simulink model "dde"  (R2015b)
settings: Solver=ode23s  StartTime=0.0  StopTime=5  RelTol=1e-3
settings Model: Creator=toni  LastModifiedBy=toni
settings DataIOCC: SaveFormat=Array  SignalLoggingSaveFormat=ModelDataLogs  OutputOption=SpecifiedOutputTimes  OutputTimes=[1,2,3,4,5]
settings OptimizationCC: ExpressionDepthLimit=2147483647
settings DebuggingCC: UnderspecifiedInitializationDetection=Classic  MergeDetectMultiDrivingBlocksExec=none  SolverPrmCheckMsg=warning  FcnCallInpInsideContextMsg=EnableAllAsWarning  StateNameClashWarn=warning
settings HardwareCC: ProdBitPerPointer=32  ProdLargestAtomicFloat=None  ProdIntDivRoundTo=Undefined  ProdEndianess=Unspecified  ProdWordSize=32  ProdHWDeviceType=32-bit Generic
settings GRTTargetCC: GeneratePreprocessorConditionals=Disable all
settings ConfigComp: CovModelRefEnable=Off  CovSFcnEnable=off

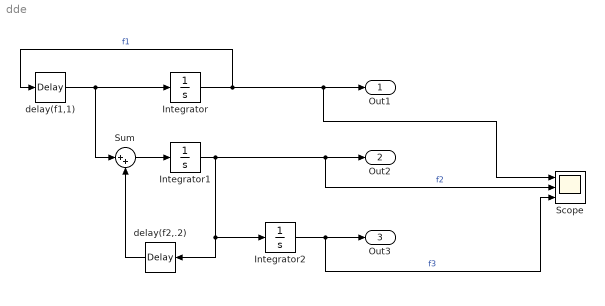
== system dde ==
  Integrator : Integrator  InitialCondition=1
  Integrator1 : Integrator  InitialCondition=1
  Integrator2 : Integrator  InitialCondition=1
  Scope : Scope  NumInputPorts=3
  Sum : Sum  Inputs=|++
  delay(f1,1) : TransportDelay  InitialOutput=1
  delay(f2,.2) : TransportDelay  DelayTime=.2  InitialOutput=1
  Out1 : Outport
  Out2 : Outport  Port=2
  Out3 : Outport  Port=3
  wires:
  delay(f1,1)/1 -> Integrator/1, Sum/1
  Integrator/1 -> delay(f1,1)/1, Out1/1, Scope/1  "f1"
  Integrator1/1 -> Scope/2, Out2/1, delay(f2,.2)/1, Integrator2/1  "f2"
  delay(f2,.2)/1 -> Sum/2
  Sum/1 -> Integrator1/1
  Integrator2/1 -> Scope/3, Out3/1  "f3"
